simulink model "transpose_core"  (R2016b)
settings: Solver=VariableStepAuto  StartTime=0.0  StopTime=512 * 64 * 3  RelTol=1e-3
model workspace (MAT data in the model file):
  dstin = [0 168430081 168430082 168430083 168430084 168430085 168430086 168430087 168430088 168430089 168430090 168430091 168430092 168430093 168430094 168430095 168430096 168430097 168430098 168430099 168430100 168430101 168430102 168430103 168430104 168430105 168430106 168430107 168430108 168430109 168430110 168430111 168430112]
  simin = [1 2 3 4 5 6 7 8 9 10 11 12 ... (294912 elements, 98304x3)]
libraries: xbsIndex_r4 x31
(part 1 of 2)
settings Model: Creator=davidm  LastModifiedBy=davidm

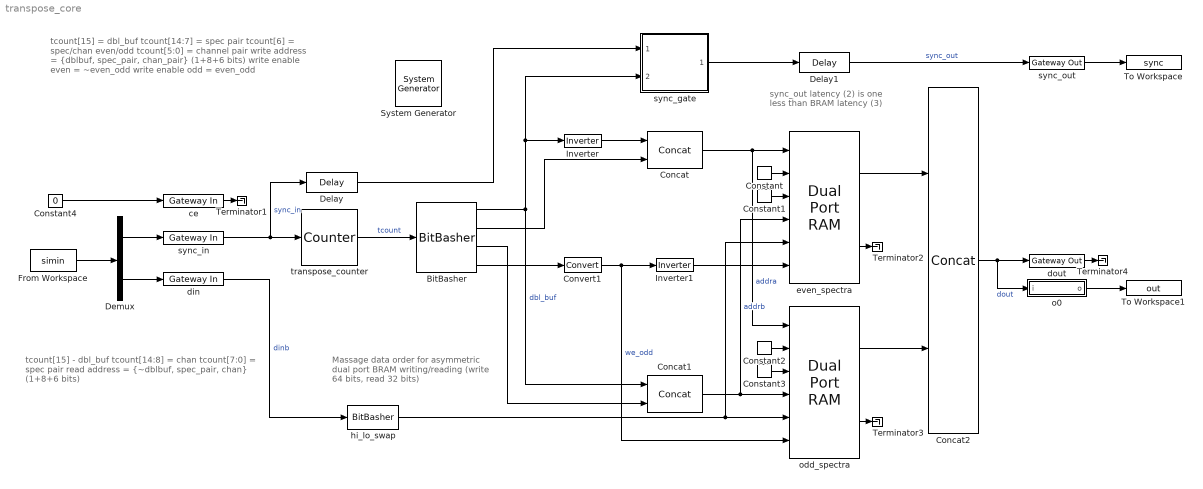
== system transpose_core ==
  note: Massage data order for asymmetric
      | dual port BRAM writing/reading
      | (write 64 bits, read 32 bits)
  note: sync_out latency (2) is one
      | less than BRAM latency (3)
  note: tcount[15] = dbl_buf
      | tcount[14:7] = spec pair
      | tcount[6] = spec/chan even/odd
      | tcount[5:0] = channel pair
      |
      | write address = {dblbuf, spec_pair, chan_pair} (1+8+6 bits)
      | write enable even = ~even_odd
      | write enable odd = even_odd
  note: tcount[15] - dbl_buf
      | tcount[14:8] = chan
      | tcount[7:0] = spec pair
      |
      | read address = {~dblbuf, spec_pair, chan} (1+8+6 bits)
  " System Generator" : xbsIndex_r4/ System Generator  Tag=genX  xilinxfamily=kintex7  part=xc7k160t  speed=-2  package=ffg676  synthesis_tool=XST  clock_wrapper=Clock Enables  directory=./transpose_core  proj_type=Project Navigator  Synth_file=XST Defaults  Impl_file=ISE Defaults  testbench=off  simulink_period=1  sysclk_period=10  dcm_input_clock_period=10  incr_netlist=off  trim_vbits=Everywhere in SubSystem  dbl_ovrd=According to Block Masks  core_generation=According to Block Masks  run_coregen=off  deprecated_control=off  eval_field=0  block_type=sysgen
  BitBasher : xbsIndex_r4/BitBasher  bitexpr=|  display_expr=off  sr_1=dbl_buf  arith_type1=Unsigned  bin_pt1=0  sr_2=rd_addr  arith_type2=Unsigned  bin_pt2=0  sr_3=wr_addr  arith_type3=Unsigned  bin_pt3=0  sr_4=we_odd  arith_type4=Unsigned  bin_pt4=0  dbl_ovrd=off  block_type=bitbasher
      | dbl_buf={in[15]}
      | rd_addr={in[7:0],in[14:8]}
      | wr_addr={in[14:7],in[5:0]}
      | we_odd={in[6]}
  Concat : xbsIndex_r4/Concat  num_inputs=2  dbl_ovrd=off  block_type=concat
  Concat1 : xbsIndex_r4/Concat  num_inputs=2  dbl_ovrd=off  block_type=concat
  Concat2 : xbsIndex_r4/Concat  num_inputs=2  dbl_ovrd=off  block_type=concat
  Constant : xbsIndex_r4/Constant  const=0  gui_display_data_type=Fixed-point  arith_type=Unsigned  n_bits=32  bin_pt=0  preci_type=Single  exp_width=8  frac_width=24  explicit_period=off  period=1  equ=P=C  opselect=C  inp2=PCIN>>17  opr=+  inp1=P  carry=CIN  dbl_ovrd=off  block_type=constant
  Constant1 : xbsIndex_r4/Constant  const=0  gui_display_data_type=Boolean  arith_type=Boolean  n_bits=16  bin_pt=14  preci_type=Single  exp_width=8  frac_width=24  explicit_period=off  period=1  equ=P=C  opselect=C  inp2=PCIN>>17  opr=+  inp1=P  carry=CIN  dbl_ovrd=off  block_type=constant
  Constant2 : xbsIndex_r4/Constant  const=0  gui_display_data_type=Fixed-point  arith_type=Unsigned  n_bits=32  bin_pt=0  preci_type=Single  exp_width=8  frac_width=24  explicit_period=off  period=1  equ=P=C  opselect=C  inp2=PCIN>>17  opr=+  inp1=P  carry=CIN  dbl_ovrd=off  block_type=constant
  Constant3 : xbsIndex_r4/Constant  const=0  gui_display_data_type=Boolean  arith_type=Boolean  n_bits=16  bin_pt=14  preci_type=Single  exp_width=8  frac_width=24  explicit_period=off  period=1  equ=P=C  opselect=C  inp2=PCIN>>17  opr=+  inp1=P  carry=CIN  dbl_ovrd=off  block_type=constant
  Constant4 : Constant  Value=0
  Convert1 : xbsIndex_r4/Convert  gui_display_data_type=Boolean  arith_type=Boolean  n_bits=16  bin_pt=14  float_type=Single  exp_bits=8  fraction_bits=24  quantization=Truncate  overflow=Wrap  en=off  latency=0  pipeline=off  dbl_ovrd=off  block_type=convert
  Delay : xbsIndex_r4/Delay  rst=off  infoeditControl=Selection of Reset will increase slice count due to use of real FFs and instead of SRLs  en=off  latency=2  reg_retiming=off  dbl_ovrd=off  block_type=delay
  Delay1 : xbsIndex_r4/Delay  rst=off  infoeditControl=Selection of Reset will increase slice count due to use of real FFs and instead of SRLs  en=off  latency=3-1  reg_retiming=off  dbl_ovrd=off  block_type=delay
  Demux : Demux  Outputs=2
  From Workspace : FromWorkspace  VariableName=simin  SampleTime=0
  Inverter : xbsIndex_r4/Inverter  en=off  latency=0  dbl_ovrd=off  block_type=inv
  Inverter1 : xbsIndex_r4/Inverter  en=off  latency=0  dbl_ovrd=off  block_type=inv
  Terminator{1..4} (4 alike) : Terminator
  To Workspace : ToWorkspace  VariableName=sync  SampleTime=-1
  To Workspace1 : ToWorkspace  VariableName=out  SampleTime=-1
  ce : xbsIndex_r4/Gateway In  gui_display_data_type=Fixed-point  arith_type=Unsigned  n_bits=1  bin_pt=0  preci_type=Single  exp_width=8  frac_width=24  rows=1  columns=1  quantization="Round  (unbiased: +/- Inf)"  overflow=Saturate  period=1  UseAsADC=off  ADCChannel='1'  interface=None  automatic_assignment=on  address_offset=hex2dec('00')  intf_name=''  intf_description=''  default_value=0  timing_constraint=None  locs_specified=off  LOCs={}  io_standard={}  inherit_from_input=off  hdl_port=on  dbl_ovrd=off  block_type=gatewayin
  din : xbsIndex_r4/Gateway In  gui_display_data_type=Fixed-point  arith_type=Unsigned  n_bits=64  bin_pt=0  preci_type=Single  exp_width=8  frac_width=24  rows=1  columns=1  quantization="Round  (unbiased: +/- Inf)"  overflow=Saturate  period=1  UseAsADC=off  ADCChannel='1'  interface=None  automatic_assignment=on  address_offset=hex2dec('00')  intf_name=''  intf_description=''  default_value=0  timing_constraint=None  locs_specified=off  LOCs={}  io_standard={}  inherit_from_input=off  hdl_port=on  dbl_ovrd=off  block_type=gatewayin
  dout : xbsIndex_r4/Gateway Out  inherit_from_input=off  hdl_port=on  rows=1  columns=1  UseAsDAC=off  DACChannel='1'  interface=None  automatic_assignment=on  address_offset=hex2dec('00')  intf_name=''  intf_description=''  timing_constraint=None  locs_specified=off  LOCs={}  io_standard={}  block_type=gatewayout
  even_spectra : xbsIndex_r4/Dual Port RAM  depth=2^16  initVector=0  distributed_mem=Block RAM  init_a=0  init_b=0  rst_a=off  rst_b=off  en_a=off  en_b=off  latency=3  write_mode_A=Read After Write  write_mode_B=Read After Write  optimize=Speed  dbl_ovrd=off  block_type=dpram
  hi_lo_swap : xbsIndex_r4/BitBasher  bitexpr=d10={d01[31:0], d01[63:32]}  display_expr=off  sr_1=d10  arith_type1=Unsigned  bin_pt1=0  sr_2=2  arith_type2=Unsigned  bin_pt2=0  sr_3=3  arith_type3=Unsigned  bin_pt3=0  sr_4=4  arith_type4=Unsigned  bin_pt4=0  dbl_ovrd=off  block_type=bitbasher
  o0 : Subsystem
  odd_spectra : xbsIndex_r4/Dual Port RAM  depth=2^16  initVector=0  distributed_mem=Block RAM  init_a=0  init_b=0  rst_a=off  rst_b=off  en_a=off  en_b=off  latency=3  write_mode_A=Read After Write  write_mode_B=Read After Write  optimize=Speed  dbl_ovrd=off  block_type=dpram
  sync_gate : Subsystem
  sync_in : xbsIndex_r4/Gateway In  gui_display_data_type=Boolean  arith_type=Boolean  n_bits=16  bin_pt=14  preci_type=Single  exp_width=8  frac_width=24  rows=1  columns=1  quantization="Round  (unbiased: +/- Inf)"  overflow=Saturate  period=1  UseAsADC=off  ADCChannel='1'  interface=None  automatic_assignment=on  address_offset=hex2dec('00')  intf_name=''  intf_description=''  default_value=0  timing_constraint=None  locs_specified=off  LOCs={}  io_standard={}  inherit_from_input=off  hdl_port=on  dbl_ovrd=off  block_type=gatewayin
  sync_out : xbsIndex_r4/Gateway Out  inherit_from_input=off  hdl_port=on  rows=1  columns=1  UseAsDAC=off  DACChannel='1'  interface=None  automatic_assignment=on  address_offset=hex2dec('00')  intf_name=''  intf_description=''  timing_constraint=None  locs_specified=off  LOCs={}  io_standard={}  block_type=gatewayout
  transpose_counter : xbsIndex_r4/Counter  cnt_type=Free Running  cnt_to=Inf  operation=Up  start_count=0  cnt_by_val=1  arith_type=Unsigned  n_bits=10+5+1  bin_pt=0  load_pin=off  rst=on  en=off  explicit_period=on  period=1  use_behavioral_HDL=off  implementation=Fabric  dbl_ovrd=off  block_type=counter
  wires:
  Constant4/1 -> ce/1
  From Workspace/1 -> Demux/1
  Demux/1 -> sync_in/1
  Demux/2 -> din/1
  sync_in/1 -> Delay/1, transpose_counter/1  "sync_in"
  transpose_counter/1 -> BitBasher/1  "tcount"
  BitBasher/2 -> Concat/2
  Inverter/1 -> Concat/1
  BitBasher/3 -> Concat1/2
  Concat1/1 -> even_spectra/4, odd_spectra/4  "addrb"
  Concat/1 -> odd_spectra/1, even_spectra/1  "addra"
  BitBasher/4 -> Convert1/1
  Inverter1/1 -> even_spectra/6
  din/1 -> hi_lo_swap/1  "dinb"
  even_spectra/1 -> Concat2/1
  odd_spectra/1 -> Concat2/2
  Concat2/1 -> o0/1(i), dout/1  "dout"
  ce/1 -> Terminator1/1
  Constant/1 -> even_spectra/2
  Constant1/1 -> even_spectra/3
  even_spectra/2 -> Terminator2/1
  Constant2/1 -> odd_spectra/2
  Constant3/1 -> odd_spectra/3
  odd_spectra/2 -> Terminator3/1
  sync_out/1 -> To Workspace/1
  o0/1(o) -> To Workspace1/1
  dout/1 -> Terminator4/1
  Convert1/1 -> odd_spectra/6, Inverter1/1  "we_odd"
  BitBasher/1 -> Concat1/1, sync_gate/2(dbl_buf), Inverter/1  "dbl_buf"
  Delay/1 -> sync_gate/1(sync_in)
  sync_gate/1(sync_out) -> Delay1/1
  Delay1/1 -> sync_out/1  "sync_out"
  hi_lo_swap/1 -> even_spectra/5, odd_spectra/5
